simulink model "BLT_filter1"  (R2020a)
settings: Solver=FixedStepAuto  StartTime=0.0  StopTime=10.0  FixedStep=0.2  RelTol=1e-3
settings Model: Creator=kiran  LastModifiedBy=kiran
settings DataIOCC: SaveOutput=off  SaveTime=off

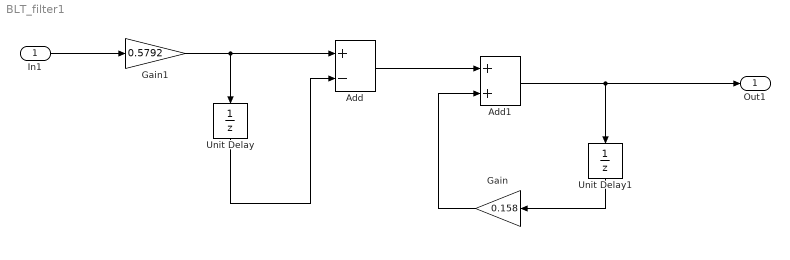
== system BLT_filter1 ==
  In1 : Inport  OutDataTypeStr=double  PortDimensions=1  SampleTime=[0.20000000000000001,0]
  Add : Sum  Inputs=+-
  Add1 : Sum
  Gain : Gain  Gain=0.158
  Gain1 : Gain  Gain=0.5792
  Unit Delay : UnitDelay  SampleTime=-1  HasFrameUpgradeWarning=on
  Unit Delay1 : UnitDelay  SampleTime=-1  HasFrameUpgradeWarning=on
  Out1 : Outport  OutDataTypeStr=double  PortDimensions=1  SampleTime=[0.20000000000000001,0]
  wires:
  In1/1 -> Gain1/1
  Unit Delay1/1 -> Gain/1
  Add1/1 -> Unit Delay1/1, Out1/1
  Add/1 -> Add1/1
  Gain1/1 -> Add/1, Unit Delay/1
  Gain/1 -> Add1/2
  Unit Delay/1 -> Add/2
